simulink model "gm_HDL_pfc_gold_fi"  (R2024b)
settings: Solver=FixedStepDiscrete  StartTime=0.0  StopTime=.4  RelTol=1e-3
InitFcn:
  | fidelity_pfc_vals;
  | load('C:\Users\Angel\Desktop\hil\pfc3ph\matlab\sim\sschdl\pfc_desktop\stateSpaceParameters.mat');
undefined symbols (not defined in the file or in its folder): a, b, c, Down, tsw, Up
libraries: hdlmdlgenlib x24, simulink x23, hdlsllib x7, eePwmGenerator x3, dspsrcs4 x3, simulink_need_slupdate x1
(part 2 of 3)

== system gm_HDL_pfc_gold_fi/simscape_system/simscape_system/FET_CTRL/crp_temp_shared ==
  in0 : Inport  OutDataTypeStr=fixdt(1, 18, 6)  PortDimensions=[6]  SampleTime=7.65403750478377e-09
  in1 : Inport  Port=2  OutDataTypeStr=fixdt(1, 18, 6)  PortDimensions=[6]  SampleTime=7.65403750478377e-09
  enb_counter : Inport  Port=3  OutDataTypeStr=fixdt(0, 7, 0)  SampleTime=7.65403750478377e-09
  Gain1 : Product  Inputs=**  OutDataTypeStr=fixdt(1, 36, 0)  SampleTime=7.65403750478377e-09
  Gain1_const : Constant  Value=-1  OutDataTypeStr=fixdt(1, 18, 17)  SampleTime=7.65403750478377e-09
  Gain3_const : Constant  Value=0.019999980926513671875  OutDataTypeStr=fixdt(1, 18, 22)  SampleTime=7.65403750478377e-09
  Gain3_out1_bypass : Subsystem
  HwModeRegister : Delay  DelayLength=double(1)  InitialCondition=0  SampleTime=7.65403750478377e-09
  HwModeRegister1 : Delay  DelayLength=double(1)  InitialCondition=0  SampleTime=7.65403750478377e-09
  PipelineRegister : Delay  DelayLength=double(1)  InitialCondition=0  SampleTime=7.65403750478377e-09
  Serializer_Subnetwork : Subsystem
  Serializer_Subnetwork1 : Subsystem
  _in0_unit_delay : simulink_need_slupdate/Unit Delay Enabled  vinit=0.0  tsamp=-1
  counter : Subsystem
  enb_counter_eq_23 : simulink/Logic and Bit Operations/Compare To Constant  relop===  const=double(23)  OutDataTypeStr=boolean
  enb_counter_eq_24 : simulink/Logic and Bit Operations/Compare To Constant  relop===  const=double(24)  OutDataTypeStr=boolean
  enb_counter_le_1 : simulink/Logic and Bit Operations/Compare To Constant  relop=<=  const=double(1)  OutDataTypeStr=boolean
  mux : Mux  Inputs=2
  mux1 : Mux  Inputs=2
  nequ_dtc{,1..3} (4 alike) : DataTypeConversion  OutDataTypeStr=fixdt(1, 18, 0)  ConvertRealWorld=Stored Integer (SI)  SampleTime=7.65403750478377e-09  SaturateOnIntegerOverflow=off  RndMeth=Floor
  nequ_dtc4 : DataTypeConversion  OutDataTypeStr=fixdt(1, 36, 23)  ConvertRealWorld=Stored Integer (SI)  SampleTime=7.65403750478377e-09  SaturateOnIntegerOverflow=off  RndMeth=Floor
  nequ_dtc5 : DataTypeConversion  OutDataTypeStr=fixdt(1, 36, 28)  ConvertRealWorld=Stored Integer (SI)  SampleTime=7.65403750478377e-09  SaturateOnIntegerOverflow=off  RndMeth=Floor
  rd_0 : Delay  DelayLength=double(10)  InitialCondition=0  SampleTime=7.65403750478377e-09
  rd_{1..2,5..6} (4 alike) : Delay  DelayLength=double(1)  InitialCondition=0  SampleTime=7.65403750478377e-09
  rd_3 : Delay  DelayLength=double(29)  InitialCondition=0  SampleTime=7.65403750478377e-09
  rd_4 : Delay  DelayLength=double(29)  InitialCondition=0  SampleTime=7.65403750478377e-09
  rd_7 : Delay  DelayLength=double(10)  InitialCondition=0  SampleTime=7.65403750478377e-09
  out0 : Outport  OutDataTypeStr=fixdt(1, 36, 23)  PortDimensions=[6]  SampleTime=7.65403750478377e-09
  out1 : Outport  Port=2  OutDataTypeStr=fixdt(1, 36, 28)  PortDimensions=[6]  SampleTime=7.65403750478377e-09
  wires:
  enb_counter/1 -> enb_counter_eq_23/1, enb_counter_eq_24/1, enb_counter_le_1/1
  enb_counter_eq_24/1 -> rd_7/1
  in0/1 -> nequ_dtc/1
  enb_counter_le_1/1 -> rd_2/1
  mux/1 -> rd_1/1
  in1/1 -> nequ_dtc1/1
  Gain1_const/1 -> nequ_dtc2/1
  Gain3_const/1 -> nequ_dtc3/1
  enb_counter_eq_23/1 -> rd_0/1
  nequ_dtc/1 -> mux/1
  nequ_dtc1/1 -> mux/2
  nequ_dtc2/1 -> mux1/1
  nequ_dtc3/1 -> mux1/2
  rd_2/1 -> counter/Enable
  PipelineRegister/1 -> rd_6/1, rd_5/1
  mux1/1 -> Serializer_Subnetwork1/1(in0)
  counter/1(out0) -> Serializer_Subnetwork1/2(in1), rd_3/1
  rd_1/1 -> Serializer_Subnetwork/1(in0)
  rd_3/1 -> Serializer_Subnetwork/2(in1)
  rd_5/1 -> _in0_unit_delay/1
  Serializer_Subnetwork1/1(out0) -> rd_4/1
  Serializer_Subnetwork/1(out0) -> HwModeRegister/1
  rd_4/1 -> HwModeRegister1/1
  HwModeRegister/1 -> Gain1/1
  HwModeRegister1/1 -> Gain1/2
  Gain1/1 -> PipelineRegister/1
  rd_0/1 -> _in0_unit_delay/2
  rd_7/1 -> Gain3_out1_bypass/2(in1)
  rd_6/1 -> Gain3_out1_bypass/1(in0)
  Gain3_out1_bypass/1(out0) -> nequ_dtc5/1
  _in0_unit_delay/1 -> nequ_dtc4/1
  nequ_dtc5/1 -> out1/1
  nequ_dtc4/1 -> out0/1

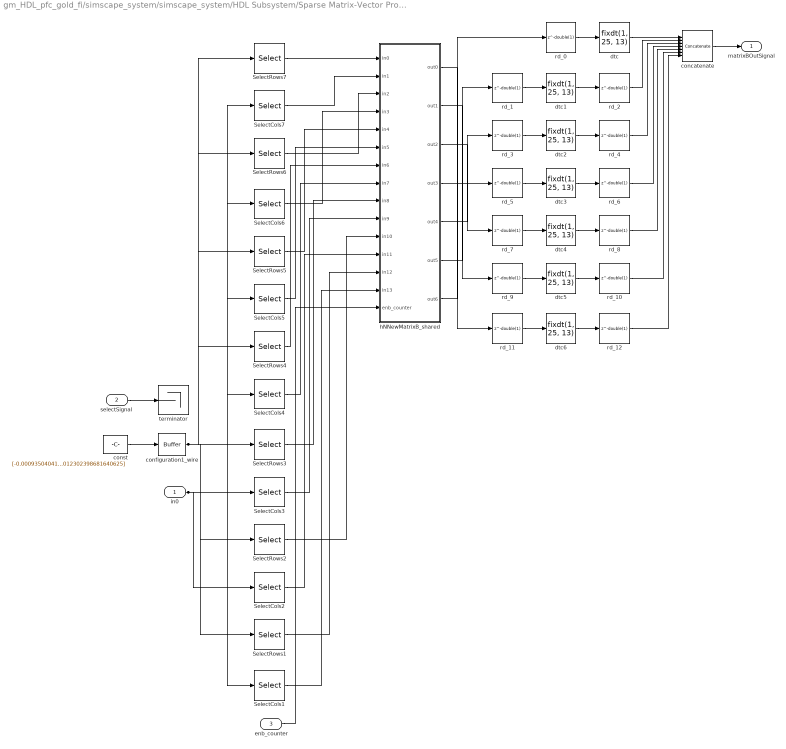
== system gm_HDL_pfc_gold_fi/simscape_system/simscape_system/HDL Subsystem/Sparse Matrix-Vector Product ==
  in0 : Inport  OutDataTypeStr=fixdt(1, 25, 13)  PortDimensions=[10]  SampleTime=7.65403750478377e-09
  selectSignal : Inport  Port=2  OutDataTypeStr=boolean  SampleTime=7.65403750478377e-09
  enb_counter : Inport  Port=3  OutDataTypeStr=fixdt(0, 7, 0)  SampleTime=7.65403750478377e-09
  SelectCols{1..6} (6 alike) : Selector  InputPortWidth=10  IndexOptions=Index vector (dialog)  Indices=double([2 3 4 5 6 7 8 9 10])  OutputSizes=double(1)
  SelectCols7 : Selector  InputPortWidth=10  IndexOptions=Index vector (dialog)  Indices=double([1 2 3 4 5 6 7 8 9])  OutputSizes=double(1)
  SelectRows1 : Selector  InputPortWidth=63  IndexOptions=Index vector (dialog)  Indices=double([2 9 16 23 30 37 44 51 58])  OutputSizes=double(1)
  SelectRows2 : Selector  InputPortWidth=63  IndexOptions=Index vector (dialog)  Indices=double([3 10 17 24 31 38 45 52 59])  OutputSizes=double(1)
  SelectRows3 : Selector  InputPortWidth=63  IndexOptions=Index vector (dialog)  Indices=double([4 11 18 25 32 39 46 53 60])  OutputSizes=double(1)
  SelectRows4 : Selector  InputPortWidth=63  IndexOptions=Index vector (dialog)  Indices=double([5 12 19 26 33 40 47 54 61])  OutputSizes=double(1)
  SelectRows5 : Selector  InputPortWidth=63  IndexOptions=Index vector (dialog)  Indices=double([6 13 20 27 34 41 48 55 62])  OutputSizes=double(1)
  SelectRows6 : Selector  InputPortWidth=63  IndexOptions=Index vector (dialog)  Indices=double([7 14 21 28 35 42 49 56 63])  OutputSizes=double(1)
  SelectRows7 : Selector  InputPortWidth=63  IndexOptions=Index vector (dialog)  Indices=double([1 8 15 22 29 36 43 50 57])  OutputSizes=double(1)
  concatenate : Concatenate  NumInputs=7
  configuration1_wire : hdlmdlgenlib/Buffer
  const : Constant  Value=[-0.000935040414333343505859375;0.00615119002759456634521484375;-0.003075595013797283172607421875;-0.003075595013797283172607421875;-0.003075600601732730865478515625;-0.003075600601732730865478515625;0.0061512016691267490386962890625;0.0004675202071666717529296875;-0.00615119002759456634521484375;0.003075595013797283172607421875;0.003075595013797283172607421875;0.003075600601732730865478515625;0.003075600601732730865478515625;-0.0061512016691267490386962890625;0.0004675202071666717529296875;0.003075595013797283172607421875;-0.00615119002759456634521484375;0.003075595013797283172607421875;-0.0061512016691267490386962890625;0.003075600601732730865478515625;0.003075600601732730865478515625;0.0004675202071666717529296875;0.003075595013797283172607421875;0.003075595013797283172607421875;-0.00615119002759456634521484375;0.003075600601732730865478515625;-0.0061512016691267490386962890625;0.003075600601732730865478515625;0.0004675202071666717529296875;-0.003075595013797283172607421875;0.00615119002759456634521484375;-0.003075595013797283172607421875;0.0061512016691267490386962890625;-0.003075600601732730865478515625;-0.003075600601732730865478515625;0.0004675202071666717529296875;-0.003075595013797283172607421875;-0.003075595013797283172607421875;0.00615119002759456634521484375;-0.003075600601732730865478515625;0.0061512016691267490386962890625;-0.003075600601732730865478515625;0.0004675202071666717529296875;0.0002460475079715251922607421875;-0.00012302398681640625;-0.00012302398681640625;-0.00012302398681640625;-0.00012302398681640625;0.0002460479736328125;0;-0.00012302398681640625;0.0002460475079715251922607421875;-0.00012302398681640625;0.0002460479736328125;-0.00012302398681640625;-0.00012302398681640625;0;-0.00012302398681640625;-0.00012302398681640625;0.0002460475079715251922607421875;-0.00012302398681640625;0.0002460479736328125;-0.00012302398681640625]  OutDataTypeStr=fixdt(1, 25, 31)  SampleTime=7.65403750478377e-09
  dtc{,1..6} (7 alike) : DataTypeConversion  OutDataTypeStr=fixdt(1, 25, 13)  RndMeth=Nearest  SampleTime=7.65403750478377e-09  SaturateOnIntegerOverflow=off
  hNNewMatrixB_shared : Subsystem
  rd_{0..12} (13 alike) : Delay  DelayLength=double(1)  InitialCondition=0  SampleTime=7.65403750478377e-09
  terminator : Terminator
  matrixBOutSignal : Outport  OutDataTypeStr=fixdt(1, 25, 13)  PortDimensions=[7]  SampleTime=7.65403750478377e-09
  wires:
  SelectCols7/1 -> hNNewMatrixB_shared/2(in1)
  SelectRows7/1 -> hNNewMatrixB_shared/1(in0)
  rd_6/1 -> concatenate/4
  selectSignal/1 -> terminator/1
  SelectRows6/1 -> hNNewMatrixB_shared/3(in2)
  in0/1 -> SelectCols5/1, SelectCols4/1, SelectCols6/1, SelectCols3/1, SelectCols7/1, SelectCols2/1, SelectCols1/1
  rd_1/1 -> dtc1/1
  const/1 -> configuration1_wire/1
  configuration1_wire/1 -> SelectRows5/1, SelectRows7/1, SelectRows4/1, SelectRows3/1, SelectRows6/1, SelectRows2/1, SelectRows1/1
  SelectCols6/1 -> hNNewMatrixB_shared/4(in3)
  hNNewMatrixB_shared/6(out5) -> rd_1/1
  SelectRows5/1 -> hNNewMatrixB_shared/5(in4)
  SelectCols5/1 -> hNNewMatrixB_shared/6(in5)
  SelectRows4/1 -> hNNewMatrixB_shared/7(in6)
  SelectCols4/1 -> hNNewMatrixB_shared/8(in7)
  SelectRows3/1 -> hNNewMatrixB_shared/9(in8)
  SelectCols3/1 -> hNNewMatrixB_shared/10(in9)
  SelectRows2/1 -> hNNewMatrixB_shared/11(in10)
  hNNewMatrixB_shared/7(out6) -> rd_0/1
  SelectCols2/1 -> hNNewMatrixB_shared/12(in11)
  dtc6/1 -> rd_12/1
  SelectRows1/1 -> hNNewMatrixB_shared/13(in12)
  SelectCols1/1 -> hNNewMatrixB_shared/14(in13)
  enb_counter/1 -> hNNewMatrixB_shared/15(enb_counter)
  hNNewMatrixB_shared/1(out0) -> rd_11/1
  hNNewMatrixB_shared/2(out1) -> rd_9/1
  hNNewMatrixB_shared/3(out2) -> rd_7/1
  hNNewMatrixB_shared/4(out3) -> rd_5/1
  hNNewMatrixB_shared/5(out4) -> rd_3/1
  rd_3/1 -> dtc2/1
  rd_11/1 -> dtc6/1
  rd_5/1 -> dtc3/1
  dtc4/1 -> rd_8/1
  rd_7/1 -> dtc4/1
  rd_9/1 -> dtc5/1
  rd_0/1 -> dtc/1
  dtc1/1 -> rd_2/1
  dtc2/1 -> rd_4/1
  dtc3/1 -> rd_6/1
  dtc5/1 -> rd_10/1
  dtc/1 -> concatenate/1
  rd_2/1 -> concatenate/2
  rd_4/1 -> concatenate/3
  concatenate/1 -> matrixBOutSignal/1
  rd_8/1 -> concatenate/5
  rd_10/1 -> concatenate/6
  rd_12/1 -> concatenate/7

== system gm_HDL_pfc_gold_fi/simscape_system/simscape_system/HDL Subsystem/Sparse Matrix-Vector Product1 ==
  delayOutSignal : Inport  OutDataTypeStr=fixdt(1, 25, 13)  PortDimensions=[7]  SampleTime=7.65403750478377e-09
  selectSignal : Inport  Port=2  OutDataTypeStr=boolean  SampleTime=7.65403750478377e-09
  enb_counter : Inport  Port=3  OutDataTypeStr=fixdt(0, 7, 0)  SampleTime=7.65403750478377e-09
  SelectCols{1..6} (6 alike) : Selector  InputPortWidth=7  IndexOptions=Index vector (dialog)  Indices=double([1 2 3 4 5 6])  OutputSizes=double(1)
  SelectCols7 : Selector  InputPortWidth=7  IndexOptions=Index vector (dialog)  Indices=double([1 2 3 4 5 7])  OutputSizes=double(1)
  SelectRows1 : Selector  InputPortWidth=42  IndexOptions=Index vector (dialog)  Indices=double([1 8 15 22 29 36])  OutputSizes=double(1)
  SelectRows2 : Selector  InputPortWidth=42  IndexOptions=Index vector (dialog)  Indices=double([2 9 16 23 30 37])  OutputSizes=double(1)
  SelectRows3 : Selector  InputPortWidth=42  IndexOptions=Index vector (dialog)  Indices=double([3 10 17 24 31 38])  OutputSizes=double(1)
  SelectRows4 : Selector  InputPortWidth=42  IndexOptions=Index vector (dialog)  Indices=double([4 11 18 25 32 39])  OutputSizes=double(1)
  SelectRows5 : Selector  InputPortWidth=42  IndexOptions=Index vector (dialog)  Indices=double([5 12 19 26 33 40])  OutputSizes=double(1)
  SelectRows6 : Selector  InputPortWidth=42  IndexOptions=Index vector (dialog)  Indices=double([6 13 20 27 34 41])  OutputSizes=double(1)
  SelectRows7 : Selector  InputPortWidth=42  IndexOptions=Index vector (dialog)  Indices=double([7 14 21 28 35 42])  OutputSizes=double(1)
  concatenate : Concatenate  NumInputs=7
  configuration1_wire : hdlmdlgenlib/Buffer
  const : Constant  Value=[0.559759318828582763671875;-0.27987849712371826171875;-0.27987849712371826171875;-0.279879033565521240234375;-0.279879033565521240234375;0.55975806713104248046875;0;-0.27987849712371826171875;0.559759318828582763671875;-0.27987849712371826171875;0.55975806713104248046875;-0.279879033565521240234375;-0.279879033565521240234375;0;-0.27987849712371826171875;-0.27987849712371826171875;0.559759318828582763671875;-0.279879033565521240234375;0.55975806713104248046875;-0.279879033565521240234375;0;-0.05037820339202880859375;0.100756466388702392578125;-0.05037820339202880859375;0.100757062435150146484375;-0.050378322601318359375;-0.050378322601318359375;0;-0.05037820339202880859375;-0.05037820339202880859375;0.100756466388702392578125;-0.050378322601318359375;0.100757062435150146484375;-0.050378322601318359375;0;0.100756466388702392578125;-0.05037820339202880859375;-0.05037820339202880859375;-0.050378322601318359375;-0.050378322601318359375;0.100757062435150146484375;0.999971926212310791015625]  OutDataTypeStr=fixdt(1, 25, 24)  SampleTime=7.65403750478377e-09
  dtc{,1..6} (7 alike) : DataTypeConversion  OutDataTypeStr=fixdt(1, 25, 13)  RndMeth=Nearest  SampleTime=7.65403750478377e-09  SaturateOnIntegerOverflow=off
  hNNewMatrixA_shared : Subsystem
  rd_{0..12} (13 alike) : Delay  DelayLength=double(1)  InitialCondition=0  SampleTime=7.65403750478377e-09
  terminator : Terminator
  matrixAOutSignal : Outport  OutDataTypeStr=fixdt(1, 25, 13)  PortDimensions=[7]  SampleTime=7.65403750478377e-09
  wires:
  SelectRows4/1 -> hNNewMatrixA_shared/7(in6)
  selectSignal/1 -> terminator/1
  configuration1_wire/1 -> SelectRows7/1, SelectRows6/1, SelectRows5/1, SelectRows2/1, SelectRows4/1, SelectRows1/1, SelectRows3/1
  dtc4/1 -> rd_8/1
  SelectCols4/1 -> hNNewMatrixA_shared/8(in7)
  const/1 -> configuration1_wire/1
  delayOutSignal/1 -> SelectCols6/1, SelectCols5/1, SelectCols7/1, SelectCols4/1, SelectCols3/1, SelectCols2/1, SelectCols1/1
  SelectRows6/1 -> hNNewMatrixA_shared/3(in2)
  dtc5/1 -> rd_10/1
  rd_5/1 -> dtc3/1
  SelectRows7/1 -> hNNewMatrixA_shared/1(in0)
  SelectCols7/1 -> hNNewMatrixA_shared/2(in1)
  SelectCols1/1 -> hNNewMatrixA_shared/14(in13)
  SelectCols6/1 -> hNNewMatrixA_shared/4(in3)
  SelectRows5/1 -> hNNewMatrixA_shared/5(in4)
  rd_0/1 -> dtc/1
  SelectCols5/1 -> hNNewMatrixA_shared/6(in5)
  SelectRows3/1 -> hNNewMatrixA_shared/9(in8)
  rd_11/1 -> dtc6/1
  SelectRows2/1 -> hNNewMatrixA_shared/11(in10)
  SelectCols3/1 -> hNNewMatrixA_shared/10(in9)
  hNNewMatrixA_shared/6(out5) -> rd_1/1
  SelectCols2/1 -> hNNewMatrixA_shared/12(in11)
  SelectRows1/1 -> hNNewMatrixA_shared/13(in12)
  enb_counter/1 -> hNNewMatrixA_shared/15(enb_counter)
  hNNewMatrixA_shared/1(out0) -> rd_11/1
  hNNewMatrixA_shared/2(out1) -> rd_9/1
  hNNewMatrixA_shared/3(out2) -> rd_7/1
  hNNewMatrixA_shared/4(out3) -> rd_5/1
  dtc/1 -> concatenate/1
  hNNewMatrixA_shared/5(out4) -> rd_3/1
  hNNewMatrixA_shared/7(out6) -> rd_0/1
  rd_1/1 -> dtc1/1
  rd_3/1 -> dtc2/1
  rd_7/1 -> dtc4/1
  rd_9/1 -> dtc5/1
  dtc1/1 -> rd_2/1
  dtc2/1 -> rd_4/1
  dtc3/1 -> rd_6/1
  dtc6/1 -> rd_12/1
  rd_2/1 -> concatenate/2
  concatenate/1 -> matrixAOutSignal/1
  rd_4/1 -> concatenate/3
  rd_6/1 -> concatenate/4
  rd_8/1 -> concatenate/5
  rd_10/1 -> concatenate/6
  rd_12/1 -> concatenate/7

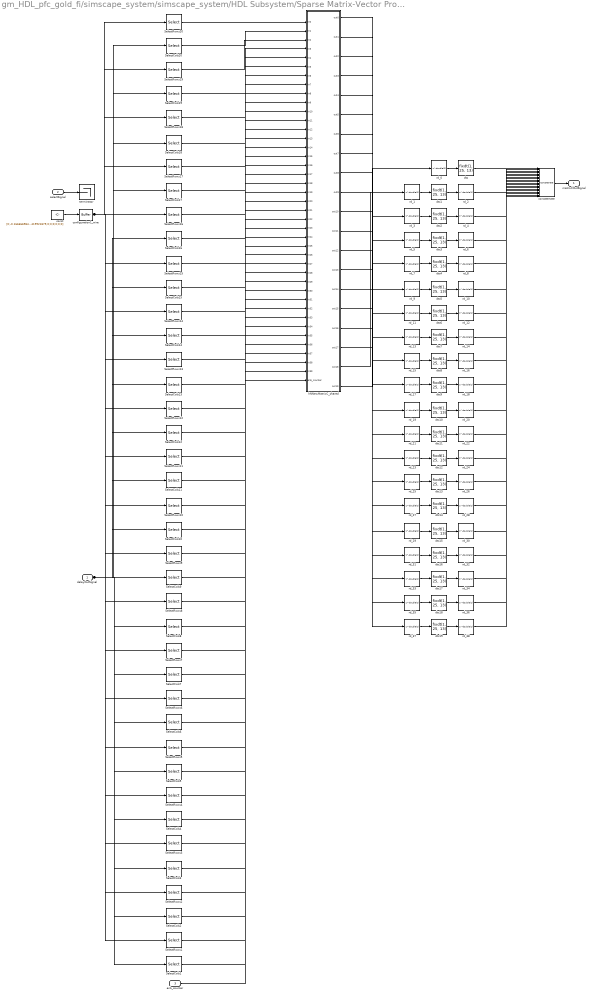
== system gm_HDL_pfc_gold_fi/simscape_system/simscape_system/HDL Subsystem/Sparse Matrix-Vector Product2 ==
  delayOutSignal : Inport  OutDataTypeStr=fixdt(1, 25, 13)  PortDimensions=[7]  SampleTime=7.65403750478377e-09
  selectSignal : Inport  Port=2  OutDataTypeStr=boolean  SampleTime=7.65403750478377e-09
  enb_counter : Inport  Port=3  OutDataTypeStr=fixdt(0, 7, 0)  SampleTime=7.65403750478377e-09
  SelectCols{1..20} (20 alike) : Selector  InputPortWidth=7  IndexOptions=Index vector (dialog)  Indices=double([1 2 3 4 5 6 7])  OutputSizes=double(1)
  SelectRows1 : Selector  InputPortWidth=140  IndexOptions=Index vector (dialog)  Indices=double([1 21 41 61 81 101 121])  OutputSizes=double(1)
  SelectRows10 : Selector  InputPortWidth=140  IndexOptions=Index vector (dialog)  Indices=double([10 30 50 70 90 110 130])  OutputSizes=double(1)
  SelectRows11 : Selector  InputPortWidth=140  IndexOptions=Index vector (dialog)  Indices=double([11 31 51 71 91 111 131])  OutputSizes=double(1)
  SelectRows12 : Selector  InputPortWidth=140  IndexOptions=Index vector (dialog)  Indices=double([12 32 52 72 92 112 132])  OutputSizes=double(1)
  SelectRows13 : Selector  InputPortWidth=140  IndexOptions=Index vector (dialog)  Indices=double([13 33 53 73 93 113 133])  OutputSizes=double(1)
  SelectRows14 : Selector  InputPortWidth=140  IndexOptions=Index vector (dialog)  Indices=double([14 34 54 74 94 114 134])  OutputSizes=double(1)
  SelectRows15 : Selector  InputPortWidth=140  IndexOptions=Index vector (dialog)  Indices=double([15 35 55 75 95 115 135])  OutputSizes=double(1)
  SelectRows16 : Selector  InputPortWidth=140  IndexOptions=Index vector (dialog)  Indices=double([16 36 56 76 96 116 136])  OutputSizes=double(1)
  SelectRows17 : Selector  InputPortWidth=140  IndexOptions=Index vector (dialog)  Indices=double([17 37 57 77 97 117 137])  OutputSizes=double(1)
  SelectRows18 : Selector  InputPortWidth=140  IndexOptions=Index vector (dialog)  Indices=double([18 38 58 78 98 118 138])  OutputSizes=double(1)
  SelectRows19 : Selector  InputPortWidth=140  IndexOptions=Index vector (dialog)  Indices=double([19 39 59 79 99 119 139])  OutputSizes=double(1)
  SelectRows2 : Selector  InputPortWidth=140  IndexOptions=Index vector (dialog)  Indices=double([2 22 42 62 82 102 122])  OutputSizes=double(1)
  SelectRows20 : Selector  InputPortWidth=140  IndexOptions=Index vector (dialog)  Indices=double([20 40 60 80 100 120 140])  OutputSizes=double(1)
  SelectRows3 : Selector  InputPortWidth=140  IndexOptions=Index vector (dialog)  Indices=double([3 23 43 63 83 103 123])  OutputSizes=double(1)
  SelectRows4 : Selector  InputPortWidth=140  IndexOptions=Index vector (dialog)  Indices=double([4 24 44 64 84 104 124])  OutputSizes=double(1)
  SelectRows5 : Selector  InputPortWidth=140  IndexOptions=Index vector (dialog)  Indices=double([5 25 45 65 85 105 125])  OutputSizes=double(1)
  SelectRows6 : Selector  InputPortWidth=140  IndexOptions=Index vector (dialog)  Indices=double([6 26 46 66 86 106 126])  OutputSizes=double(1)
  SelectRows7 : Selector  InputPortWidth=140  IndexOptions=Index vector (dialog)  Indices=double([7 27 47 67 87 107 127])  OutputSizes=double(1)
  SelectRows8 : Selector  InputPortWidth=140  IndexOptions=Index vector (dialog)  Indices=double([8 28 48 68 88 108 128])  OutputSizes=double(1)
  SelectRows9 : Selector  InputPortWidth=140  IndexOptions=Index vector (dialog)  Indices=double([9 29 49 69 89 109 129])  OutputSizes=double(1)
  concatenate : Concatenate  NumInputs=20
  configuration1_wire : hdlmdlgenlib/Buffer
  const : Constant  Value=[0;-0.16666698455810546875;-8.33333301544189453125;0.16666698455810546875;8.33333301544189453125;-0.08333301544189453125;-4.1666660308837890625;-0.08333301544189453125;-4.16666698455810546875;0.08333301544189453125;4.16666698455810546875;0.08333301544189453125;4.16666698455810546875;0;-0.16666698455810546875;-0.16666698455810546875;0.33333301544189453125;0;0;0;0;0.08333301544189453125;4.16666698455810546875;-0.08333301544189453125;-4.1666660308837890625;0.16666698455810546875;8.33333301544189453125;-0.08333301544189453125;-4.16666698455810546875;-0.16666698455810546875;-8.33333301544189453125;0.08333301544189453125;4.16666698455810546875;0;0.33333301544189453125;-0.16666698455810546875;-0.16666698455810546875;0;0;0;0;0.08333301544189453125;4.16666698455810546875;-0.08333301544189453125;-4.16666698455810546875;-0.08333301544189453125;-4.16666698455810546875;0.16666698455810546875;8.33333301544189453125;0.08333301544189453125;4.16666698455810546875;-0.16666698455810546875;-8.33333301544189453125;0;-0.16666698455810546875;0.33333301544189453125;-0.16666698455810546875;0;0;0;0;0.08333301544189453125;4.16666698455810546875;-0.08333301544189453125;-4.1666660308837890625;0.16666698455810546875;8.33333301544189453125;-0.08333301544189453125;-4.16666698455810546875;-0.16666698455810546875;-8.33333301544189453125;0.08333301544189453125;4.16666698455810546875;0;0.33333301544189453125;-0.16666698455810546875;-0.16666698455810546875;0;0;0;0;0.08333301544189453125;4.16666698455810546875;-0.08333301544189453125;-4.16666698455810546875;-0.08333301544189453125;-4.16666698455810546875;0.16666698455810546875;8.33333301544189453125;0.08333301544189453125;4.16666698455810546875;-0.16666698455810546875;-8.33333301544189453125;0;-0.16666698455810546875;0.33333301544189453125;-0.16666698455810546875;0;0;0;0;-0.16666698455810546875;-8.33333301544189453125;0.16666698455810546875;8.33333301544189453125;-0.08333301544189453125;-4.16666698455810546875;-0.08333301544189453125;-4.16666698455810546875;0.08333301544189453125;4.16666698455810546875;0.08333301544189453125;4.16666698455810546875;0;-0.16666698455810546875;-0.16666698455810546875;0.33333301544189453125;0;0;0;0;0.009998321533203125;0.4999103546142578125;0.009998321533203125;0.4999103546142578125;0.009998321533203125;0.4999103546142578125;0.009998321533203125;0.4999103546142578125;0.009998321533203125;0.4999103546142578125;0.009998321533203125;0.4999103546142578125;0.99981975555419921875;0;0;0;0;0;0]  OutDataTypeStr=fixdt(1, 25, 20)  SampleTime=7.65403750478377e-09
  dtc{,1..19} (20 alike) : DataTypeConversion  OutDataTypeStr=fixdt(1, 25, 13)  RndMeth=Nearest  SampleTime=7.65403750478377e-09  SaturateOnIntegerOverflow=off
  hNNewMatrixC_shared : Subsystem
  rd_{0..38} (39 alike) : Delay  DelayLength=double(1)  InitialCondition=0  SampleTime=7.65403750478377e-09
  terminator : Terminator
  matrixCOutSignal : Outport  OutDataTypeStr=fixdt(1, 25, 13)  PortDimensions=[20]  SampleTime=7.65403750478377e-09
  wires:
  rd_38/1 -> concatenate/20
  hNNewMatrixC_shared/4(out3) -> rd_31/1
  rd_34/1 -> concatenate/18
  dtc8/1 -> rd_16/1
  rd_6/1 -> concatenate/4
  configuration1_wire/1 -> SelectRows19/1, SelectRows18/1, SelectRows16/1, SelectRows14/1, SelectRows11/1, SelectRows9/1, SelectRows8/1, SelectRows7/1, SelectRows6/1, SelectRows4/1, SelectRows3/1, SelectRows1/1, SelectRows5/1, SelectRows10/1, SelectRows20/1, SelectRows15/1, SelectRows2/1, SelectRows13/1, SelectRows17/1, SelectRows12/1
  SelectCols12/1 -> hNNewMatrixC_shared/18(in17)
  dtc18/1 -> rd_36/1
  rd_28/1 -> concatenate/15
  SelectRows18/1 -> hNNewMatrixC_shared/5(in4)
  rd_18/1 -> concatenate/10
  rd_27/1 -> dtc14/1
  rd_21/1 -> dtc11/1
  rd_2/1 -> concatenate/2
  SelectCols1/1 -> hNNewMatrixC_shared/40(in39)
  rd_22/1 -> concatenate/12
  rd_36/1 -> concatenate/19
  rd_24/1 -> concatenate/13
  rd_32/1 -> concatenate/17
  SelectCols17/1 -> hNNewMatrixC_shared/8(in7)
  rd_30/1 -> concatenate/16
  rd_25/1 -> dtc13/1
  rd_11/1 -> dtc6/1
  SelectRows1/1 -> hNNewMatrixC_shared/39(in38)
  rd_33/1 -> dtc17/1
  rd_5/1 -> dtc3/1
  SelectRows9/1 -> hNNewMatrixC_shared/23(in22)
  rd_4/1 -> concatenate/3
  rd_26/1 -> concatenate/14
  rd_31/1 -> dtc16/1
  SelectRows7/1 -> hNNewMatrixC_shared/27(in26)
  rd_35/1 -> dtc18/1
  SelectRows3/1 -> hNNewMatrixC_shared/35(in34)
  rd_20/1 -> concatenate/11
  rd_8/1 -> concatenate/5
  rd_3/1 -> dtc2/1
  rd_16/1 -> concatenate/9
  rd_9/1 -> dtc5/1
  rd_14/1 -> concatenate/8
  rd_23/1 -> dtc12/1
  SelectRows16/1 -> hNNewMatrixC_shared/9(in8)
  rd_12/1 -> concatenate/7
  dtc4/1 -> rd_8/1
  delayOutSignal/1 -> SelectCols20/1, SelectCols19/1, SelectCols18/1, SelectCols17/1, SelectCols16/1, SelectCols14/1, SelectCols13/1, SelectCols12/1, SelectCols8/1, SelectCols6/1, SelectCols5/1, SelectCols2/1, SelectCols1/1, SelectCols7/1, SelectCols4/1, SelectCols15/1, SelectCols3/1, SelectCols11/1, SelectCols10/1, SelectCols9/1
  dtc17/1 -> rd_34/1
  rd_17/1 -> dtc9/1
  hNNewMatrixC_shared/2(out1) -> rd_35/1
  rd_10/1 -> concatenate/6
  dtc13/1 -> rd_26/1
  hNNewMatrixC_shared/19(out18) -> rd_1/1
  dtc14/1 -> rd_28/1
  rd_0/1 -> dtc/1
  dtc12/1 -> rd_24/1
  rd_1/1 -> dtc1/1
  rd_13/1 -> dtc7/1
  rd_7/1 -> dtc4/1
  rd_15/1 -> dtc8/1
  dtc9/1 -> rd_18/1
  rd_19/1 -> dtc10/1
  dtc16/1 -> rd_32/1
  dtc19/1 -> rd_38/1
  rd_29/1 -> dtc15/1
  hNNewMatrixC_shared/1(out0) -> rd_37/1
  dtc15/1 -> rd_30/1
  SelectRows12/1 -> hNNewMatrixC_shared/17(in16)
  dtc10/1 -> rd_20/1
  rd_37/1 -> dtc19/1
  enb_counter/1 -> hNNewMatrixC_shared/41(enb_counter)
  SelectCols10/1 -> hNNewMatrixC_shared/22(in21)
  dtc7/1 -> rd_14/1
  dtc11/1 -> rd_22/1
  dtc6/1 -> rd_12/1
  dtc5/1 -> rd_10/1
  SelectCols14/1 -> hNNewMatrixC_shared/14(in13)
  dtc3/1 -> rd_6/1
  dtc2/1 -> rd_4/1
  SelectRows2/1 -> hNNewMatrixC_shared/37(in36)
  hNNewMatrixC_shared/14(out13) -> rd_11/1
  dtc1/1 -> rd_2/1
  dtc/1 -> concatenate/1
  hNNewMatrixC_shared/3(out2) -> rd_33/1
  hNNewMatrixC_shared/5(out4) -> rd_29/1
  hNNewMatrixC_shared/6(out5) -> rd_27/1
  hNNewMatrixC_shared/7(out6) -> rd_25/1
  hNNewMatrixC_shared/8(out7) -> rd_23/1
  hNNewMatrixC_shared/9(out8) -> rd_21/1
  hNNewMatrixC_shared/10(out9) -> rd_19/1
  hNNewMatrixC_shared/11(out10) -> rd_17/1
  hNNewMatrixC_shared/12(out11) -> rd_15/1
  hNNewMatrixC_shared/13(out12) -> rd_13/1
  hNNewMatrixC_shared/15(out14) -> rd_9/1
  hNNewMatrixC_shared/16(out15) -> rd_7/1
  hNNewMatrixC_shared/17(out16) -> rd_5/1
  SelectCols7/1 -> hNNewMatrixC_shared/28(in27)
  hNNewMatrixC_shared/18(out17) -> rd_3/1
  SelectCols20/1 -> hNNewMatrixC_shared/2(in1)
  SelectCols19/1 -> hNNewMatrixC_shared/4(in3)
  SelectCols18/1 -> hNNewMatrixC_shared/6(in5)
  SelectCols9/1 -> hNNewMatrixC_shared/24(in23)
  SelectCols16/1 -> hNNewMatrixC_shared/10(in9)
  SelectCols15/1 -> hNNewMatrixC_shared/12(in11)
  SelectCols13/1 -> hNNewMatrixC_shared/16(in15)
  SelectCols11/1 -> hNNewMatrixC_shared/20(in19)
  SelectRows19/1 -> hNNewMatrixC_shared/3(in2)
  SelectCols8/1 -> hNNewMatrixC_shared/26(in25)
  SelectCols6/1 -> hNNewMatrixC_shared/30(in29)
  SelectCols5/1 -> hNNewMatrixC_shared/32(in31)
  SelectCols4/1 -> hNNewMatrixC_shared/34(in33)
  SelectCols3/1 -> hNNewMatrixC_shared/36(in35)
  SelectCols2/1 -> hNNewMatrixC_shared/38(in37)
  SelectRows20/1 -> hNNewMatrixC_shared/1(in0)
  SelectRows17/1 -> hNNewMatrixC_shared/7(in6)
  SelectRows15/1 -> hNNewMatrixC_shared/11(in10)
  SelectRows14/1 -> hNNewMatrixC_shared/13(in12)
  SelectRows13/1 -> hNNewMatrixC_shared/15(in14)
  SelectRows11/1 -> hNNewMatrixC_shared/19(in18)
  SelectRows10/1 -> hNNewMatrixC_shared/21(in20)
  SelectRows8/1 -> hNNewMatrixC_shared/25(in24)
  SelectRows6/1 -> hNNewMatrixC_shared/29(in28)
  SelectRows5/1 -> hNNewMatrixC_shared/31(in30)
  SelectRows4/1 -> hNNewMatrixC_shared/33(in32)
  const/1 -> configuration1_wire/1
  concatenate/1 -> matrixCOutSignal/1
  selectSignal/1 -> terminator/1
  hNNewMatrixC_shared/20(out19) -> rd_0/1

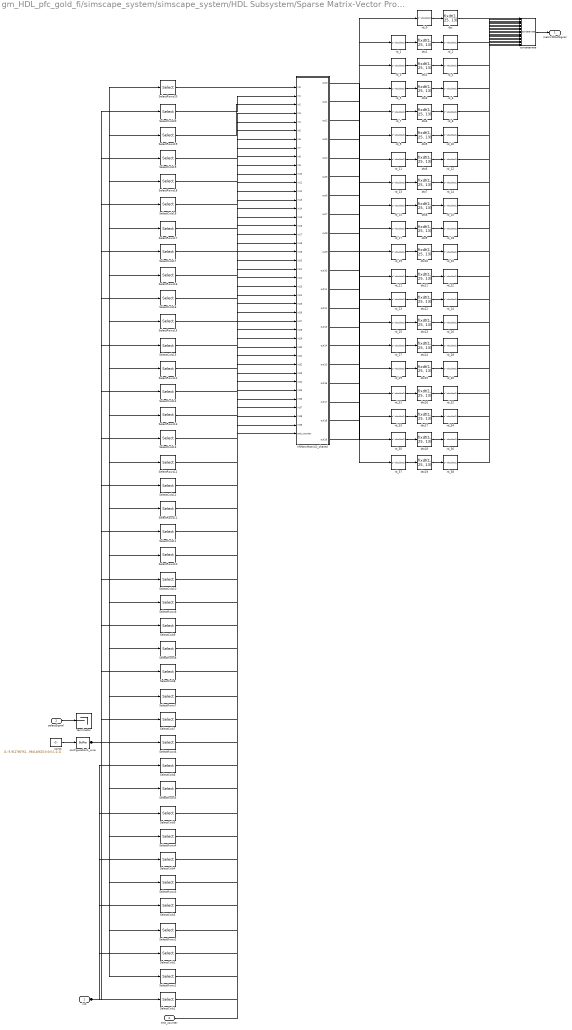
== system gm_HDL_pfc_gold_fi/simscape_system/simscape_system/HDL Subsystem/Sparse Matrix-Vector Product3 ==
  in0 : Inport  OutDataTypeStr=fixdt(1, 25, 13)  PortDimensions=[10]  SampleTime=7.65403750478377e-09
  selectSignal : Inport  Port=2  OutDataTypeStr=boolean  SampleTime=7.65403750478377e-09
  enb_counter : Inport  Port=3  OutDataTypeStr=fixdt(0, 7, 0)  SampleTime=7.65403750478377e-09
  SelectCols{1..17} (17 alike) : Selector  InputPortWidth=10  IndexOptions=Index vector (dialog)  Indices=double([1 2 3 4 5 6 7])  OutputSizes=double(1)
  SelectCols18 : Selector  InputPortWidth=10  IndexOptions=Index vector (dialog)  Indices=double([1 2 3 4 5 6 9])  OutputSizes=double(1)
  SelectCols19 : Selector  InputPortWidth=10  IndexOptions=Index vector (dialog)  Indices=double([1 2 3 4 5 6 10])  OutputSizes=double(1)
  SelectCols20 : Selector  InputPortWidth=10  IndexOptions=Index vector (dialog)  Indices=double([1 2 3 4 5 6 8])  OutputSizes=double(1)
  SelectRows1 : Selector  InputPortWidth=140  IndexOptions=Index vector (dialog)  Indices=double([1 21 41 61 81 101 121])  OutputSizes=double(1)
  SelectRows10 : Selector  InputPortWidth=140  IndexOptions=Index vector (dialog)  Indices=double([10 30 50 70 90 110 130])  OutputSizes=double(1)
  SelectRows11 : Selector  InputPortWidth=140  IndexOptions=Index vector (dialog)  Indices=double([11 31 51 71 91 111 131])  OutputSizes=double(1)
  SelectRows12 : Selector  InputPortWidth=140  IndexOptions=Index vector (dialog)  Indices=double([12 32 52 72 92 112 132])  OutputSizes=double(1)
  SelectRows13 : Selector  InputPortWidth=140  IndexOptions=Index vector (dialog)  Indices=double([13 33 53 73 93 113 133])  OutputSizes=double(1)
  SelectRows14 : Selector  InputPortWidth=140  IndexOptions=Index vector (dialog)  Indices=double([14 34 54 74 94 114 134])  OutputSizes=double(1)
  SelectRows15 : Selector  InputPortWidth=140  IndexOptions=Index vector (dialog)  Indices=double([15 35 55 75 95 115 135])  OutputSizes=double(1)
  SelectRows16 : Selector  InputPortWidth=140  IndexOptions=Index vector (dialog)  Indices=double([16 36 56 76 96 116 136])  OutputSizes=double(1)
  SelectRows17 : Selector  InputPortWidth=140  IndexOptions=Index vector (dialog)  Indices=double([17 37 57 77 97 117 137])  OutputSizes=double(1)
  SelectRows18 : Selector  InputPortWidth=140  IndexOptions=Index vector (dialog)  Indices=double([18 38 58 78 98 118 139])  OutputSizes=double(1)
  SelectRows19 : Selector  InputPortWidth=140  IndexOptions=Index vector (dialog)  Indices=double([19 39 59 79 99 119 140])  OutputSizes=double(1)
  SelectRows2 : Selector  InputPortWidth=140  IndexOptions=Index vector (dialog)  Indices=double([2 22 42 62 82 102 122])  OutputSizes=double(1)
  SelectRows20 : Selector  InputPortWidth=140  IndexOptions=Index vector (dialog)  Indices=double([20 40 60 80 100 120 138])  OutputSizes=double(1)
  SelectRows3 : Selector  InputPortWidth=140  IndexOptions=Index vector (dialog)  Indices=double([3 23 43 63 83 103 123])  OutputSizes=double(1)
  SelectRows4 : Selector  InputPortWidth=140  IndexOptions=Index vector (dialog)  Indices=double([4 24 44 64 84 104 124])  OutputSizes=double(1)
  SelectRows5 : Selector  InputPortWidth=140  IndexOptions=Index vector (dialog)  Indices=double([5 25 45 65 85 105 125])  OutputSizes=double(1)
  SelectRows6 : Selector  InputPortWidth=140  IndexOptions=Index vector (dialog)  Indices=double([6 26 46 66 86 106 126])  OutputSizes=double(1)
  SelectRows7 : Selector  InputPortWidth=140  IndexOptions=Index vector (dialog)  Indices=double([7 27 47 67 87 107 127])  OutputSizes=double(1)
  SelectRows8 : Selector  InputPortWidth=140  IndexOptions=Index vector (dialog)  Indices=double([8 28 48 68 88 108 128])  OutputSizes=double(1)
  SelectRows9 : Selector  InputPortWidth=140  IndexOptions=Index vector (dialog)  Indices=double([9 29 49 69 89 109 129])  OutputSizes=double(1)
  concatenate : Concatenate  NumInputs=20
  configuration1_wire : hdlmdlgenlib/Buffer
  const : Constant  Value=[1;-5.91278076171875e-05;-0.0030002593994140625;-5.91278076171875e-05;-0.0030002593994140625;-5.91278076171875e-05;-0.0030002593994140625;-5.91278076171875e-05;-0.0030002593994140625;-5.91278076171875e-05;-0.0030002593994140625;-5.91278076171875e-05;-0.0030002593994140625;-0.0059986114501953125;0;0;0;0;0;0;0;-0.499969482421875;25.001499176025390625;-0.499969482421875;-24.998500823974609375;3.0517578125e-05;0.001499176025390625;3.0517578125e-05;0.001499176025390625;3.0517578125e-05;0.001499176025390625;3.0517578125e-05;0.001499176025390625;0.0030002593994140625;0;0;0;0;0;0;0;-0.499969482421875;-24.998500823974609375;-0.499969482421875;25.001499176025390625;3.0517578125e-05;0.001499176025390625;3.0517578125e-05;0.001499176025390625;3.0517578125e-05;0.001499176025390625;3.0517578125e-05;0.001499176025390625;0.0030002593994140625;0;0;0;0;0;0;0;3.0517578125e-05;0.001499176025390625;3.0517578125e-05;0.001499176025390625;-0.499969482421875;25.001499176025390625;3.0517578125e-05;0.001499176025390625;-0.499969482421875;-24.998500823974609375;3.0517578125e-05;0.001499176025390625;0.0030002593994140625;0;0;0;0;0;0;0;3.0517578125e-05;0.001499176025390625;3.0517578125e-05;0.001499176025390625;3.0517578125e-05;0.001499176025390625;-0.499969482421875;25.001499176025390625;3.0517578125e-05;0.001499176025390625;-0.499969482421875;-24.998500823974609375;0.0030002593994140625;0;0;0;0;0;0;0;3.0517578125e-05;0.001499176025390625;3.0517578125e-05;0.001499176025390625;-0.499969482421875;-24.998500823974609375;3.0517578125e-05;0.001499176025390625;-0.499969482421875;25.001499176025390625;3.0517578125e-05;0.001499176025390625;0.0030002593994140625;0;0;0;0;0;0;0;3.0517578125e-05;0.001499176025390625;3.0517578125e-05;0.001499176025390625;3.0517578125e-05;0.001499176025390625;-0.499969482421875;-24.998500823974609375;3.0517578125e-05;0.001499176025390625;-0.499969482421875;25.001499176025390625;0.0030002593994140625;0;0;0;1;1;1]  OutDataTypeStr=fixdt(1, 25, 19)  SampleTime=7.65403750478377e-09
  dtc{,1..19} (20 alike) : DataTypeConversion  OutDataTypeStr=fixdt(1, 25, 13)  RndMeth=Nearest  SampleTime=7.65403750478377e-09  SaturateOnIntegerOverflow=off
  hNNewMatrixD_shared : Subsystem
  rd_{0..38} (39 alike) : Delay  DelayLength=double(1)  InitialCondition=0  SampleTime=7.65403750478377e-09
  terminator : Terminator
  matrixDOutSignal : Outport  OutDataTypeStr=fixdt(1, 25, 13)  PortDimensions=[20]  SampleTime=7.65403750478377e-09
  wires:
  SelectRows2/1 -> hNNewMatrixD_shared/37(in36)
  rd_38/1 -> concatenate/20
  SelectCols17/1 -> hNNewMatrixD_shared/8(in7)
  rd_22/1 -> concatenate/12
  rd_7/1 -> dtc4/1
  rd_30/1 -> concatenate/16
  SelectRows1/1 -> hNNewMatrixD_shared/39(in38)
  dtc6/1 -> rd_12/1
  rd_16/1 -> concatenate/9
  hNNewMatrixD_shared/13(out12) -> rd_13/1
  rd_36/1 -> concatenate/19
  hNNewMatrixD_shared/10(out9) -> rd_19/1
  rd_14/1 -> concatenate/8
  rd_24/1 -> concatenate/13
  dtc9/1 -> rd_18/1
  rd_17/1 -> dtc9/1
  dtc3/1 -> rd_6/1
  rd_26/1 -> concatenate/14
  dtc/1 -> concatenate/1
  dtc11/1 -> rd_22/1
  rd_34/1 -> concatenate/18
  dtc17/1 -> rd_34/1
  rd_27/1 -> dtc14/1
  rd_5/1 -> dtc3/1
  rd_11/1 -> dtc6/1
  dtc10/1 -> rd_20/1
  hNNewMatrixD_shared/18(out17) -> rd_3/1
  rd_32/1 -> concatenate/17
  rd_9/1 -> dtc5/1
  rd_28/1 -> concatenate/15
  rd_20/1 -> concatenate/11
  enb_counter/1 -> hNNewMatrixD_shared/41(enb_counter)
  dtc7/1 -> rd_14/1
  hNNewMatrixD_shared/19(out18) -> rd_1/1
  rd_2/1 -> concatenate/2
  rd_18/1 -> concatenate/10
  dtc15/1 -> rd_30/1
  in0/1 -> SelectCols18/1, SelectCols17/1, SelectCols16/1, SelectCols14/1, SelectCols13/1, SelectCols12/1, SelectCols10/1, SelectCols9/1, SelectCols11/1, SelectCols8/1, SelectCols7/1, SelectCols6/1, SelectCols5/1, SelectCols4/1, SelectCols2/1, SelectCols1/1, SelectCols19/1, SelectCols15/1, SelectCols3/1, SelectCols20/1
  dtc2/1 -> rd_4/1
  SelectCols10/1 -> hNNewMatrixD_shared/22(in21)
  rd_33/1 -> dtc17/1
  rd_12/1 -> concatenate/7
  SelectRows12/1 -> hNNewMatrixD_shared/17(in16)
  dtc5/1 -> rd_10/1
  rd_21/1 -> dtc11/1
  rd_10/1 -> concatenate/6
  rd_8/1 -> concatenate/5
  SelectRows14/1 -> hNNewMatrixD_shared/13(in12)
  dtc12/1 -> rd_24/1
  rd_23/1 -> dtc12/1
  rd_0/1 -> dtc/1
  rd_31/1 -> dtc16/1
  rd_6/1 -> concatenate/4
  SelectCols9/1 -> hNNewMatrixD_shared/24(in23)
  rd_19/1 -> dtc10/1
  rd_3/1 -> dtc2/1
  rd_4/1 -> concatenate/3
  dtc18/1 -> rd_36/1
  SelectRows8/1 -> hNNewMatrixD_shared/25(in24)
  hNNewMatrixD_shared/3(out2) -> rd_33/1
  rd_29/1 -> dtc15/1
  rd_25/1 -> dtc13/1
  hNNewMatrixD_shared/12(out11) -> rd_15/1
  rd_35/1 -> dtc18/1
  rd_13/1 -> dtc7/1
  rd_1/1 -> dtc1/1
  rd_37/1 -> dtc19/1
  rd_15/1 -> dtc8/1
  dtc14/1 -> rd_28/1
  SelectRows13/1 -> hNNewMatrixD_shared/15(in14)
  dtc19/1 -> rd_38/1
  dtc16/1 -> rd_32/1
  dtc13/1 -> rd_26/1
  hNNewMatrixD_shared/1(out0) -> rd_37/1
  dtc8/1 -> rd_16/1
  dtc4/1 -> rd_8/1
  dtc1/1 -> rd_2/1
  hNNewMatrixD_shared/2(out1) -> rd_35/1
  hNNewMatrixD_shared/4(out3) -> rd_31/1
  SelectCols18/1 -> hNNewMatrixD_shared/6(in5)
  hNNewMatrixD_shared/5(out4) -> rd_29/1
  SelectCols19/1 -> hNNewMatrixD_shared/4(in3)
  hNNewMatrixD_shared/6(out5) -> rd_27/1
  hNNewMatrixD_shared/7(out6) -> rd_25/1
  hNNewMatrixD_shared/8(out7) -> rd_23/1
  hNNewMatrixD_shared/9(out8) -> rd_21/1
  hNNewMatrixD_shared/11(out10) -> rd_17/1
  SelectCols1/1 -> hNNewMatrixD_shared/40(in39)
  configuration1_wire/1 -> SelectRows20/1, SelectRows19/1, SelectRows17/1, SelectRows16/1, SelectRows15/1, SelectRows14/1, SelectRows13/1, SelectRows12/1, SelectRows10/1, SelectRows7/1, SelectRows6/1, SelectRows5/1, SelectRows4/1, SelectRows3/1, SelectRows1/1, SelectRows8/1, SelectRows9/1, SelectRows18/1, SelectRows11/1, SelectRows2/1
  SelectRows6/1 -> hNNewMatrixD_shared/29(in28)
  hNNewMatrixD_shared/14(out13) -> rd_11/1
  hNNewMatrixD_shared/15(out14) -> rd_9/1
  hNNewMatrixD_shared/16(out15) -> rd_7/1
  SelectRows16/1 -> hNNewMatrixD_shared/9(in8)
  hNNewMatrixD_shared/17(out16) -> rd_5/1
  SelectCols20/1 -> hNNewMatrixD_shared/2(in1)
  SelectCols12/1 -> hNNewMatrixD_shared/18(in17)
  SelectCols16/1 -> hNNewMatrixD_shared/10(in9)
  SelectCols15/1 -> hNNewMatrixD_shared/12(in11)
  SelectCols14/1 -> hNNewMatrixD_shared/14(in13)
  SelectCols13/1 -> hNNewMatrixD_shared/16(in15)
  SelectCols11/1 -> hNNewMatrixD_shared/20(in19)
  SelectCols8/1 -> hNNewMatrixD_shared/26(in25)
  SelectCols7/1 -> hNNewMatrixD_shared/28(in27)
  SelectCols6/1 -> hNNewMatrixD_shared/30(in29)
  SelectCols5/1 -> hNNewMatrixD_shared/32(in31)
  SelectCols4/1 -> hNNewMatrixD_shared/34(in33)
  SelectCols3/1 -> hNNewMatrixD_shared/36(in35)
  SelectCols2/1 -> hNNewMatrixD_shared/38(in37)
  SelectRows20/1 -> hNNewMatrixD_shared/1(in0)
  SelectRows19/1 -> hNNewMatrixD_shared/3(in2)
  SelectRows18/1 -> hNNewMatrixD_shared/5(in4)
  SelectRows17/1 -> hNNewMatrixD_shared/7(in6)
  SelectRows15/1 -> hNNewMatrixD_shared/11(in10)
  SelectRows11/1 -> hNNewMatrixD_shared/19(in18)
  SelectRows10/1 -> hNNewMatrixD_shared/21(in20)
  SelectRows9/1 -> hNNewMatrixD_shared/23(in22)
  SelectRows7/1 -> hNNewMatrixD_shared/27(in26)
  SelectRows5/1 -> hNNewMatrixD_shared/31(in30)
  SelectRows4/1 -> hNNewMatrixD_shared/33(in32)
  SelectRows3/1 -> hNNewMatrixD_shared/35(in34)
  const/1 -> configuration1_wire/1
  concatenate/1 -> matrixDOutSignal/1
  selectSignal/1 -> terminator/1
  hNNewMatrixD_shared/20(out19) -> rd_0/1

== system gm_HDL_pfc_gold_fi/simscape_system/simscape_system/FET_CTRL/crp_temp_shared/Gain3_out1_bypass ==
  in0 : Inport  OutDataTypeStr=fixdt(1, 36, 0)  PortDimensions=[6]  SampleTime=7.65403750478377e-09
  in1 : Inport  Port=2  OutDataTypeStr=boolean  SampleTime=7.65403750478377e-09
  Gain3_out1_enb : Switch  Criteria=u2 ~= 0  Threshold=double(0)  OutDataTypeStr=fixdt(1, 36, 0)  SampleTime=7.65403750478377e-09  SaturateOnIntegerOverflow=off  InputSameDT=off
  Gain3_out1_state : Delay  DelayLength=double(1)  InitialCondition=0  SampleTime=7.65403750478377e-09
  out0 : Outport  OutDataTypeStr=fixdt(1, 36, 0)  PortDimensions=[6]  SampleTime=7.65403750478377e-09
  wires:
  in0/1 -> Gain3_out1_enb/1
  Gain3_out1_enb/1 -> Gain3_out1_state/1, out0/1
  in1/1 -> Gain3_out1_enb/2
  Gain3_out1_state/1 -> Gain3_out1_enb/3

== system gm_HDL_pfc_gold_fi/simscape_system/simscape_system/FET_CTRL/crp_temp_shared/Serializer_Subnetwork ==
  in0 : Inport  OutDataTypeStr=fixdt(1, 18, 0)  PortDimensions=[12]  SampleTime=7.65403750478377e-09
  in1 : Inport  Port=2  OutDataTypeStr=fixdt(0, 1, 0)  SampleTime=7.65403750478377e-09
  ratechange_splitcomp : Demux  Outputs=2
  splitcomp_multiport : MultiPortSwitch  DataPortOrder=Zero-based contiguous  Inputs=2  DiagnosticForDefault=None  zeroidx=on  OutDataTypeStr=fixdt(1, 18, 0)  SampleTime=7.65403750478377e-09  SaturateOnIntegerOverflow=off  InputSameDT=off
  out0 : Outport  OutDataTypeStr=fixdt(1, 18, 0)  PortDimensions=[6]  SampleTime=7.65403750478377e-09
  wires:
  in0/1 -> ratechange_splitcomp/1
  ratechange_splitcomp/2 -> splitcomp_multiport/3
  in1/1 -> splitcomp_multiport/1
  ratechange_splitcomp/1 -> splitcomp_multiport/2
  splitcomp_multiport/1 -> out0/1

== system gm_HDL_pfc_gold_fi/simscape_system/simscape_system/FET_CTRL/crp_temp_shared/Serializer_Subnetwork1 ==
  in0 : Inport  OutDataTypeStr=fixdt(1, 18, 0)  PortDimensions=[2]  SampleTime=7.65403750478377e-09
  in1 : Inport  Port=2  OutDataTypeStr=fixdt(0, 1, 0)  SampleTime=7.65403750478377e-09
  ratechange_splitcomp : Demux  Outputs=2
  splitcomp_multiport : MultiPortSwitch  DataPortOrder=Zero-based contiguous  Inputs=2  DiagnosticForDefault=None  zeroidx=on  OutDataTypeStr=fixdt(1, 18, 0)  SampleTime=7.65403750478377e-09  SaturateOnIntegerOverflow=off  InputSameDT=off
  out0 : Outport  OutDataTypeStr=fixdt(1, 18, 0)  SampleTime=7.65403750478377e-09
  wires:
  in1/1 -> splitcomp_multiport/1
  in0/1 -> ratechange_splitcomp/1
  ratechange_splitcomp/1 -> splitcomp_multiport/2
  ratechange_splitcomp/2 -> splitcomp_multiport/3
  splitcomp_multiport/1 -> out0/1

== system gm_HDL_pfc_gold_fi/simscape_system/simscape_system/FET_CTRL/crp_temp_shared/counter ==
  globalSchedule : EnablePort  OutDataTypeStr=boolean
  ctr_0_1 : hdlsllib/Sources/HDL Counter  CountType=Count limited  CountInit=double(0)  CountStep=double(1)  CountMax=double(1)  CountFromType=Initial value  CountFrom=double(0)  CountResetPort=off  CountLoadPort=off  CountEnbPort=off  CountDirPort=off  CountHitOutputPort=off  CountDataType=Unsigned  CountWordLen=1  CountFracLen=0  CountSampTime=7.65403750478377e-09
  out0 : Outport  OutDataTypeStr=fixdt(0, 1, 0)  SampleTime=7.65403750478377e-09  InitialOutput=0
  wires:
  ctr_0_1/1 -> out0/1

== system gm_HDL_pfc_gold_fi/simscape_system/simscape_system/HDL Subsystem/Sparse Matrix-Vector Product/hNNewMatrixB_shared ==
  in0 : Inport  OutDataTypeStr=fixdt(1, 25, 31)  PortDimensions=[9]  SampleTime=7.65403750478377e-09
  in1 : Inport  Port=2  OutDataTypeStr=fixdt(1, 25, 13)  PortDimensions=[9]  SampleTime=7.65403750478377e-09
  in2 : Inport  Port=3  OutDataTypeStr=fixdt(1, 25, 31)  PortDimensions=[9]  SampleTime=7.65403750478377e-09
  in3 : Inport  Port=4  OutDataTypeStr=fixdt(1, 25, 13)  PortDimensions=[9]  SampleTime=7.65403750478377e-09
  in4 : Inport  Port=5  OutDataTypeStr=fixdt(1, 25, 31)  PortDimensions=[9]  SampleTime=7.65403750478377e-09
  in5 : Inport  Port=6  OutDataTypeStr=fixdt(1, 25, 13)  PortDimensions=[9]  SampleTime=7.65403750478377e-09
  in6 : Inport  Port=7  OutDataTypeStr=fixdt(1, 25, 31)  PortDimensions=[9]  SampleTime=7.65403750478377e-09
  in7 : Inport  Port=8  OutDataTypeStr=fixdt(1, 25, 13)  PortDimensions=[9]  SampleTime=7.65403750478377e-09
  in8 : Inport  Port=9  OutDataTypeStr=fixdt(1, 25, 31)  PortDimensions=[9]  SampleTime=7.65403750478377e-09
  in9 : Inport  Port=10  OutDataTypeStr=fixdt(1, 25, 13)  PortDimensions=[9]  SampleTime=7.65403750478377e-09
  in10 : Inport  Port=11  OutDataTypeStr=fixdt(1, 25, 31)  PortDimensions=[9]  SampleTime=7.65403750478377e-09
  in11 : Inport  Port=12  OutDataTypeStr=fixdt(1, 25, 13)  PortDimensions=[9]  SampleTime=7.65403750478377e-09
  in12 : Inport  Port=13  OutDataTypeStr=fixdt(1, 25, 31)  PortDimensions=[9]  SampleTime=7.65403750478377e-09
  in13 : Inport  Port=14  OutDataTypeStr=fixdt(1, 25, 13)  PortDimensions=[9]  SampleTime=7.65403750478377e-09
  enb_counter : Inport  Port=15  OutDataTypeStr=fixdt(0, 7, 0)  SampleTime=7.65403750478377e-09
  Serializer_Subnetwork : Subsystem
  Serializer_Subnetwork1 : Subsystem
  counter : Subsystem
  demux : Demux  Outputs=6
  dot_product1_bypass : Subsystem
  dot_product_9 : Subsystem
  enb_counter_eq_8 : simulink/Logic and Bit Operations/Compare To Constant  relop===  const=double(8)  OutDataTypeStr=boolean
  enb_counter_ge_2 : simulink/Logic and Bit Operations/Compare To Constant  relop=>=  const=double(2)  OutDataTypeStr=boolean
  enb_counter_ge_2_and_enb_counter_le_7 : Logic  AllPortsSameDT=off  OutDataTypeStr=boolean  SampleTime=7.65403750478377e-09
  enb_counter_le_6 : simulink/Logic and Bit Operations/Compare To Constant  relop=<=  const=double(6)  OutDataTypeStr=boolean
  enb_counter_le_7 : simulink/Logic and Bit Operations/Compare To Constant  relop=<=  const=double(7)  OutDataTypeStr=boolean
  mux : Mux  Inputs=7
  mux1 : Mux  Inputs=7
  rd_{0..2,4} (4 alike) : Delay  DelayLength=double(1)  InitialCondition=0  SampleTime=7.65403750478377e-09
  rd_3 : Delay  DelayLength=double(4)  InitialCondition=0  SampleTime=7.65403750478377e-09
  rd_5 : Delay  DelayLength=double(6)  InitialCondition=0  SampleTime=7.65403750478377e-09
  tappedDelay : Subsystem
  out0 : Outport  OutDataTypeStr=fixdt(1, 50, 44)  SampleTime=7.65403750478377e-09
  out1 : Outport  Port=2  OutDataTypeStr=fixdt(1, 50, 44)  SampleTime=7.65403750478377e-09
  out2 : Outport  Port=3  OutDataTypeStr=fixdt(1, 50, 44)  SampleTime=7.65403750478377e-09
  out3 : Outport  Port=4  OutDataTypeStr=fixdt(1, 50, 44)  SampleTime=7.65403750478377e-09
  out4 : Outport  Port=5  OutDataTypeStr=fixdt(1, 50, 44)  SampleTime=7.65403750478377e-09
  out5 : Outport  Port=6  OutDataTypeStr=fixdt(1, 50, 44)  SampleTime=7.65403750478377e-09
  out6 : Outport  Port=7  OutDataTypeStr=fixdt(1, 50, 44)  SampleTime=7.65403750478377e-09
  wires:
  enb_counter_eq_8/1 -> rd_5/1
  demux/1 -> out0/1
  enb_counter/1 -> enb_counter_eq_8/1, enb_counter_ge_2/1, enb_counter_le_7/1, enb_counter_le_6/1
  counter/1(out0) -> Serializer_Subnetwork1/2(in1), Serializer_Subnetwork/2(in1)
  rd_1/1 -> enb_counter_ge_2_and_enb_counter_le_7/1
  enb_counter_ge_2/1 -> rd_1/1
  enb_counter_le_6/1 -> rd_0/1
  in0/1 -> mux/1
  demux/4 -> out3/1
  in7/1 -> mux1/4
  enb_counter_le_7/1 -> rd_2/1
  rd_2/1 -> enb_counter_ge_2_and_enb_counter_le_7/2
  in2/1 -> mux/2
  in4/1 -> mux/3
  Serializer_Subnetwork/1(out0) -> dot_product_9/1(in1)
  in6/1 -> mux/4
  dot_product1_bypass/1(out0) -> out6/1
  tappedDelay/1(out0) -> demux/1
  in8/1 -> mux/5
  in10/1 -> mux/6
  demux/6 -> out5/1
  in12/1 -> mux/7
  rd_0/1 -> counter/Enable
  in1/1 -> mux1/1
  in3/1 -> mux1/2
  in5/1 -> mux1/3
  rd_5/1 -> dot_product1_bypass/2(in1)
  in9/1 -> mux1/5
  in11/1 -> mux1/6
  in13/1 -> mux1/7
  enb_counter_ge_2_and_enb_counter_le_7/1 -> rd_3/1
  mux/1 -> Serializer_Subnetwork/1(in0)
  mux1/1 -> Serializer_Subnetwork1/1(in0)
  Serializer_Subnetwork1/1(out0) -> dot_product_9/2(in2)
  rd_3/1 -> tappedDelay/Enable
  dot_product_9/1(out1) -> rd_4/1, tappedDelay/1(in0)
  rd_4/1 -> dot_product1_bypass/1(in0)
  demux/2 -> out1/1
  demux/5 -> out4/1
  demux/3 -> out2/1

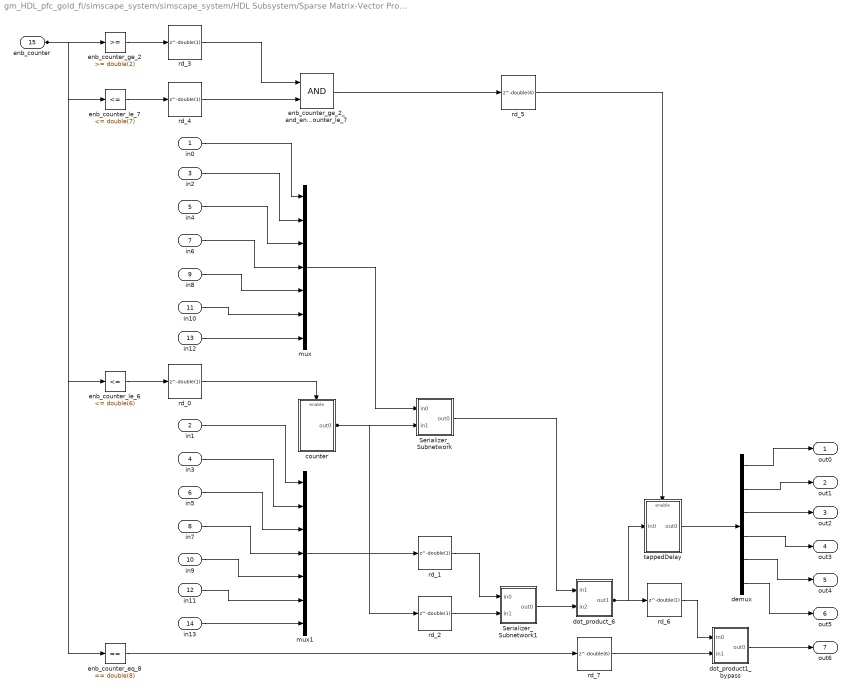
== system gm_HDL_pfc_gold_fi/simscape_system/simscape_system/HDL Subsystem/Sparse Matrix-Vector Product1/hNNewMatrixA_shared ==
  in0 : Inport  OutDataTypeStr=fixdt(1, 25, 24)  PortDimensions=[6]  SampleTime=7.65403750478377e-09
  in1 : Inport  Port=2  OutDataTypeStr=fixdt(1, 25, 13)  PortDimensions=[6]  SampleTime=7.65403750478377e-09
  in2 : Inport  Port=3  OutDataTypeStr=fixdt(1, 25, 24)  PortDimensions=[6]  SampleTime=7.65403750478377e-09
  in3 : Inport  Port=4  OutDataTypeStr=fixdt(1, 25, 13)  PortDimensions=[6]  SampleTime=7.65403750478377e-09
  in4 : Inport  Port=5  OutDataTypeStr=fixdt(1, 25, 24)  PortDimensions=[6]  SampleTime=7.65403750478377e-09
  in5 : Inport  Port=6  OutDataTypeStr=fixdt(1, 25, 13)  PortDimensions=[6]  SampleTime=7.65403750478377e-09
  in6 : Inport  Port=7  OutDataTypeStr=fixdt(1, 25, 24)  PortDimensions=[6]  SampleTime=7.65403750478377e-09
  in7 : Inport  Port=8  OutDataTypeStr=fixdt(1, 25, 13)  PortDimensions=[6]  SampleTime=7.65403750478377e-09
  in8 : Inport  Port=9  OutDataTypeStr=fixdt(1, 25, 24)  PortDimensions=[6]  SampleTime=7.65403750478377e-09
  in9 : Inport  Port=10  OutDataTypeStr=fixdt(1, 25, 13)  PortDimensions=[6]  SampleTime=7.65403750478377e-09
  in10 : Inport  Port=11  OutDataTypeStr=fixdt(1, 25, 24)  PortDimensions=[6]  SampleTime=7.65403750478377e-09
  in11 : Inport  Port=12  OutDataTypeStr=fixdt(1, 25, 13)  PortDimensions=[6]  SampleTime=7.65403750478377e-09
  in12 : Inport  Port=13  OutDataTypeStr=fixdt(1, 25, 24)  PortDimensions=[6]  SampleTime=7.65403750478377e-09
  in13 : Inport  Port=14  OutDataTypeStr=fixdt(1, 25, 13)  PortDimensions=[6]  SampleTime=7.65403750478377e-09
  enb_counter : Inport  Port=15  OutDataTypeStr=fixdt(0, 7, 0)  SampleTime=7.65403750478377e-09
  Serializer_Subnetwork : Subsystem
  Serializer_Subnetwork1 : Subsystem
  counter : Subsystem
  demux : Demux  Outputs=6
  dot_product1_bypass : Subsystem
  dot_product_6 : Subsystem
  enb_counter_eq_8 : simulink/Logic and Bit Operations/Compare To Constant  relop===  const=double(8)  OutDataTypeStr=boolean
  enb_counter_ge_2 : simulink/Logic and Bit Operations/Compare To Constant  relop=>=  const=double(2)  OutDataTypeStr=boolean
  enb_counter_ge_2_and_enb_counter_le_7 : Logic  AllPortsSameDT=off  OutDataTypeStr=boolean  SampleTime=7.65403750478377e-09
  enb_counter_le_6 : simulink/Logic and Bit Operations/Compare To Constant  relop=<=  const=double(6)  OutDataTypeStr=boolean
  enb_counter_le_7 : simulink/Logic and Bit Operations/Compare To Constant  relop=<=  const=double(7)  OutDataTypeStr=boolean
  mux : Mux  Inputs=7
  mux1 : Mux  Inputs=7
  rd_{0..4,6} (6 alike) : Delay  DelayLength=double(1)  InitialCondition=0  SampleTime=7.65403750478377e-09
  rd_5 : Delay  DelayLength=double(4)  InitialCondition=0  SampleTime=7.65403750478377e-09
  rd_7 : Delay  DelayLength=double(6)  InitialCondition=0  SampleTime=7.65403750478377e-09
  tappedDelay : Subsystem
  out0 : Outport  OutDataTypeStr=fixdt(1, 50, 37)  SampleTime=7.65403750478377e-09
  out1 : Outport  Port=2  OutDataTypeStr=fixdt(1, 50, 37)  SampleTime=7.65403750478377e-09
  out2 : Outport  Port=3  OutDataTypeStr=fixdt(1, 50, 37)  SampleTime=7.65403750478377e-09
  out3 : Outport  Port=4  OutDataTypeStr=fixdt(1, 50, 37)  SampleTime=7.65403750478377e-09
  out4 : Outport  Port=5  OutDataTypeStr=fixdt(1, 50, 37)  SampleTime=7.65403750478377e-09
  out5 : Outport  Port=6  OutDataTypeStr=fixdt(1, 50, 37)  SampleTime=7.65403750478377e-09
  out6 : Outport  Port=7  OutDataTypeStr=fixdt(1, 50, 37)  SampleTime=7.65403750478377e-09
  wires:
  dot_product_6/1(out1) -> rd_6/1, tappedDelay/1(in0)
  mux/1 -> Serializer_Subnetwork/1(in0)
  enb_counter/1 -> enb_counter_eq_8/1, enb_counter_ge_2/1, enb_counter_le_6/1, enb_counter_le_7/1
  enb_counter_le_7/1 -> rd_4/1
  demux/4 -> out3/1
  enb_counter_ge_2/1 -> rd_3/1
  rd_3/1 -> enb_counter_ge_2_and_enb_counter_le_7/1
  enb_counter_le_6/1 -> rd_0/1
  in6/1 -> mux/4
  enb_counter_eq_8/1 -> rd_7/1
  in0/1 -> mux/1
  rd_4/1 -> enb_counter_ge_2_and_enb_counter_le_7/2
  in2/1 -> mux/2
  in4/1 -> mux/3
  dot_product1_bypass/1(out0) -> out6/1
  in8/1 -> mux/5
  in10/1 -> mux/6
  in9/1 -> mux1/5
  in12/1 -> mux/7
  rd_0/1 -> counter/Enable
  rd_6/1 -> dot_product1_bypass/1(in0)
  in1/1 -> mux1/1
  in3/1 -> mux1/2
  in5/1 -> mux1/3
  in7/1 -> mux1/4
  in11/1 -> mux1/6
  demux/6 -> out5/1
  in13/1 -> mux1/7
  demux/3 -> out2/1
  enb_counter_ge_2_and_enb_counter_le_7/1 -> rd_5/1
  counter/1(out0) -> rd_2/1, Serializer_Subnetwork/2(in1)
  mux1/1 -> rd_1/1
  Serializer_Subnetwork/1(out0) -> dot_product_6/1(in1)
  rd_1/1 -> Serializer_Subnetwork1/1(in0)
  rd_2/1 -> Serializer_Subnetwork1/2(in1)
  rd_5/1 -> tappedDelay/Enable
  Serializer_Subnetwork1/1(out0) -> dot_product_6/2(in2)
  rd_7/1 -> dot_product1_bypass/2(in1)
  tappedDelay/1(out0) -> demux/1
  demux/1 -> out0/1
  demux/2 -> out1/1
  demux/5 -> out4/1
